simulink model "Pendulo_fuzzy_Comparacion_Man_Sugmatlabv2014"  (R2014a)
settings: Solver=ode4  StartTime=0.0  StopTime=10  FixedStep=0.001  MinStep=0.0000001  RelTol=1e-3
undefined symbols (not defined in the file or in its folder): evalfis, PenduloMan, PenduloSug
libraries: fuzblock x2
settings Model: Creator=posgrado  LastModifiedBy=Jesus
settings DataIOCC: SignalLoggingSaveFormat=ModelDataLogs  SignalLoggingName=sigsOut
settings OptimizationCC: BooleanDataType=off  ExpressionDepthLimit=2147483647  InitFltsAndDblsToZero=on
settings DebuggingCC: SaveWithParameterizedLinksMsg=none  UnderspecifiedInitializationDetection=Classic  SignalResolutionControl=TryResolveAllWithWarning  SolverPrmCheckMsg=none  MultiTaskDSMMsg=warning  MultiTaskCondExecSysMsg=none  FcnCallInpInsideContextMsg=UseLocalSettings  StateNameClashWarn=warning
settings HardwareCC: TargetUnknown=on
settings RTWCC: IncludeERTFirstTime=on
settings GRTTargetCC: TargetFcnLib=ansi_tfl_tmw.mat  CombineOutputUpdateFcns=off  GRTInterface=on

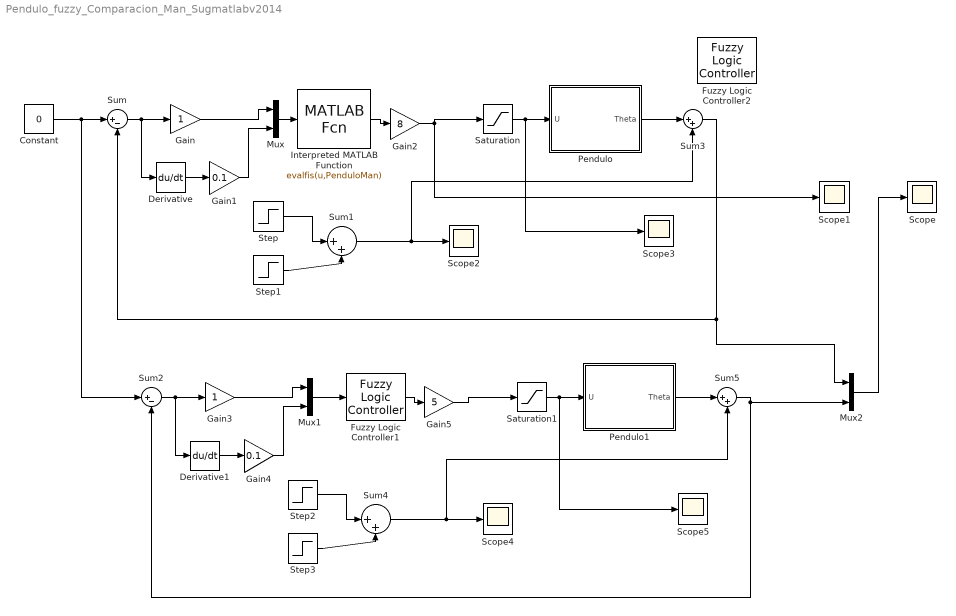
== system Pendulo_fuzzy_Comparacion_Man_Sugmatlabv2014 ==
  Constant : Constant  Value=0
  Derivative : Derivative
  Derivative1 : Derivative
  Fuzzy Logic Controller1 : fuzblock/Fuzzy Logic  Controller  fis=[PenduloSug]
  Fuzzy Logic Controller2 : fuzblock/Fuzzy Logic  Controller  fis=[PenduloMan]
  Gain : Gain
  Gain1 : Gain  Gain=0.1
  Gain2 : Gain  Gain=8
  Gain3 : Gain
  Gain4 : Gain  Gain=0.1
  Gain5 : Gain  Gain=5
  Interpreted MATLAB Function : MATLABFcn  MATLABFcn=evalfis(u,PenduloMan)
  Mux : Mux  Inputs=2
  Mux1 : Mux  Inputs=2
  Mux2 : Mux  Inputs=2
  Pendulo : Subsystem
  Pendulo1 : Subsystem
  Saturation : Saturate  UpperLimit=10  LowerLimit=-10
  Saturation1 : Saturate  UpperLimit=10  LowerLimit=-10
  Scope{,1..5} (6 alike) : Scope
      Scope settings: TimeRange=10  YMin=-0.4  YMax=0.25  MaxDataPoints=50000
      Scope1 settings: TimeRange=10  YMin=-15  YMax=10  MaxDataPoints=50000
      Scope2 settings: TimeRange=10  YMin=-1  YMax=1  SaveName=ScopeData2  MaxDataPoints=50000
      Scope3 settings: TimeRange=100  YMin=0.055  YMax=0.1  SaveName=ScopeData3  MaxDataPoints=50000
      Scope4 settings: TimeRange=10  YMin=-1  YMax=1  SaveName=ScopeData4  MaxDataPoints=50000
      Scope5 settings: TimeRange=100  YMin=0.055  YMax=0.1  SaveName=ScopeData5  MaxDataPoints=50000
  Step : Step  Time=4  After=0.2  SampleTime=0
  Step1 : Step  Time=5  After=-0.2  SampleTime=0
  Step2 : Step  Time=4  After=0.2  SampleTime=0
  Step3 : Step  Time=5  After=-0.2  SampleTime=0
  Sum : Sum  Inputs=|+-
  Sum{1,3..5} (4 alike) : Sum  Inputs=|++
  Sum2 : Sum  Inputs=|+-
  wires:
  Sum/1 -> Gain/1, Derivative/1
  Gain/1 -> Mux/1
  Mux/1 -> Interpreted MATLAB Function/1
  Interpreted MATLAB Function/1 -> Gain2/1
  Gain2/1 -> Scope1/1, Saturation/1
  Derivative/1 -> Gain1/1
  Gain1/1 -> Mux/2
  Saturation/1 -> Scope3/1, Pendulo/1(U)
  Step/1 -> Sum1/1
  Step1/1 -> Sum1/2
  Sum1/1 -> Sum3/2, Scope2/1
  Pendulo/1(Theta) -> Sum3/1
  Sum3/1 -> Mux2/1, Sum/2
  Constant/1 -> Sum2/1, Sum/1
  Sum2/1 -> Derivative1/1, Gain3/1
  Gain3/1 -> Mux1/1
  Mux1/1 -> Fuzzy Logic Controller1/1
  Fuzzy Logic Controller1/1 -> Gain5/1
  Gain5/1 -> Saturation1/1
  Derivative1/1 -> Gain4/1
  Gain4/1 -> Mux1/2
  Saturation1/1 -> Pendulo1/1(U), Scope5/1
  Step2/1 -> Sum4/1
  Step3/1 -> Sum4/2
  Sum4/1 -> Scope4/1, Sum5/2
  Pendulo1/1(Theta) -> Sum5/1
  Sum5/1 -> Mux2/2, Sum2/2
  Mux2/1 -> Scope/1

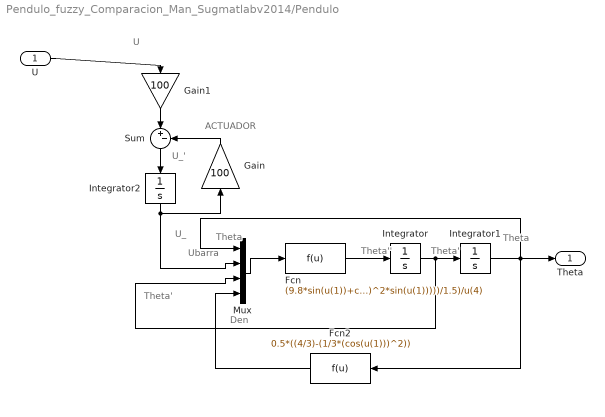
== system Pendulo_fuzzy_Comparacion_Man_Sugmatlabv2014/Pendulo ==
  note: Theta'
  note: Theta
  note: Theta''
  note: Theta
  note: U
  note: Ubarra
  note: Theta'
  note: Den
  note: U_'
  note: U_
  note: ACTUADOR
  U : Inport
  Fcn : Fcn  Expr=(9.8*sin(u(1))+cos(u(1))*(((-u(2)-0.25*u(3)^2*sin(u(1)))))/1.5)/u(4)
  Fcn2 : Fcn  Expr=0.5*((4/3)-(1/3*(cos(u(1)))^2))
  Gain : Gain  Gain=100  SaturateOnIntegerOverflow=on  OutDataTypeStr=Inherit: Same as input  ParamDataTypeStr=Inherit: Same as input
  Gain1 : Gain  Gain=100  SaturateOnIntegerOverflow=on  OutDataTypeStr=Inherit: Same as input  ParamDataTypeStr=Inherit: Same as input
  Integrator : Integrator
  Integrator1 : Integrator  InitialCondition=0.2
  Integrator2 : Integrator  InitialCondition=0.01
  Mux : Mux
  Sum : Sum  Inputs=|+-  SaturateOnIntegerOverflow=on  InputSameDT=on  OutDataTypeStr=Inherit: Same as first input
  Theta : Outport
  wires:
  Fcn/1 -> Integrator/1
  Mux/1 -> Fcn/1
  Integrator/1 -> Integrator1/1, Mux/3
  Integrator1/1 -> Mux/1, Theta/1, Fcn2/1
  Integrator2/1 -> Gain/1, Mux/2
  Sum/1 -> Integrator2/1
  Gain1/1 -> Sum/1
  Gain/1 -> Sum/2
  U/1 -> Gain1/1
  Fcn2/1 -> Mux/4

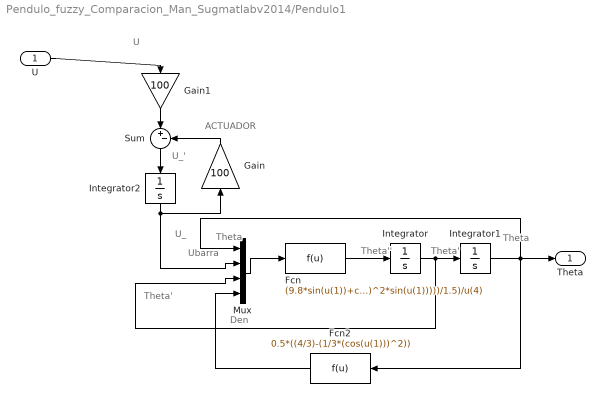
== system Pendulo_fuzzy_Comparacion_Man_Sugmatlabv2014/Pendulo1 ==
  note: ACTUADOR
  note: U_
  note: U_'
  note: Den
  note: Theta'
  note: Ubarra
  note: U
  note: Theta
  note: Theta''
  note: Theta
  note: Theta'
  U : Inport
  Fcn : Fcn  Expr=(9.8*sin(u(1))+cos(u(1))*(((-u(2)-0.25*u(3)^2*sin(u(1)))))/1.5)/u(4)
  Fcn2 : Fcn  Expr=0.5*((4/3)-(1/3*(cos(u(1)))^2))
  Gain : Gain  Gain=100  SaturateOnIntegerOverflow=on  OutDataTypeStr=Inherit: Same as input  ParamDataTypeStr=Inherit: Same as input
  Gain1 : Gain  Gain=100  SaturateOnIntegerOverflow=on  OutDataTypeStr=Inherit: Same as input  ParamDataTypeStr=Inherit: Same as input
  Integrator : Integrator
  Integrator1 : Integrator  InitialCondition=0.2
  Integrator2 : Integrator  InitialCondition=0.01
  Mux : Mux
  Sum : Sum  Inputs=|+-  SaturateOnIntegerOverflow=on  InputSameDT=on  OutDataTypeStr=Inherit: Same as first input
  Theta : Outport
  wires:
  Fcn2/1 -> Mux/4
  U/1 -> Gain1/1
  Gain/1 -> Sum/2
  Gain1/1 -> Sum/1
  Sum/1 -> Integrator2/1
  Integrator2/1 -> Mux/2, Gain/1
  Integrator1/1 -> Fcn2/1, Theta/1, Mux/1
  Integrator/1 -> Mux/3, Integrator1/1
  Mux/1 -> Fcn/1
  Fcn/1 -> Integrator/1
